simulink model "model"  (R2019b)
settings: Solver=VariableStepAuto  StartTime=0.0  StopTime=50  RelTol=1e-3
values from neighbouring files (symbols this model uses):
  k = 1    [FODT.m]
  kp = T_FODT/(2*k*T_o)    [FODT.m]
  T1 = 5    [FODT.m]
  T2 = 0.1    [FODT.m]
  T3 = 0.05    [FODT.m]
  T4 = 0.025    [FODT.m]
  T_zaklocenia = 25    [FODT.m]
  Ti = T_FODT    [FODT.m]
libraries: simulink_extras x4, simulink x1
settings Model: Creator=szymo  LastModifiedBy=szymo
settings SFSimCC: CustomCodeUndefinedFunction=UseInterfaceOnly

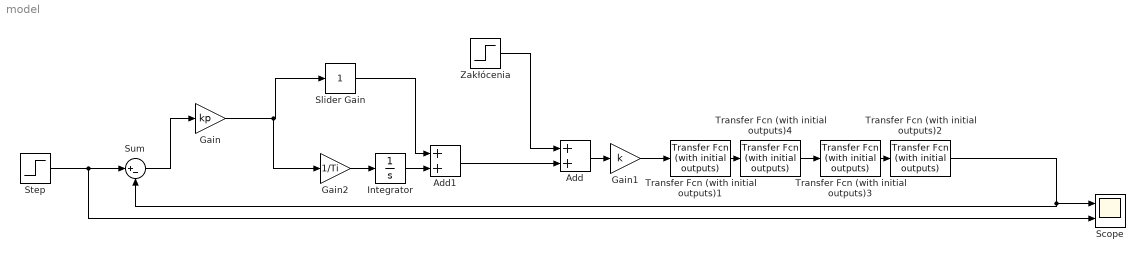
== system model ==
  Add : Sum
  Add1 : Sum
  Gain : Gain  Gain=kp
  Gain1 : Gain  Gain=k
  Gain2 : Gain  Gain=1/Ti
  Integrator : Integrator
  Scope : Scope  NumInputPorts=2
  Slider Gain : simulink/Math Operations/Slider Gain  gain=1  low=0  high=2
  Step : Step  SampleTime=0
  Sum : Sum  Inputs=|+-
  Transfer Fcn (with initial outputs)1 : simulink_extras/Additional Linear/Transfer Fcn (with initial outputs)  N=[1]  D=[T1 1]  Y0=0  U0=0
  Transfer Fcn (with initial outputs)2 : simulink_extras/Additional Linear/Transfer Fcn (with initial outputs)  N=[1]  D="[T4  1]"  Y0=0  U0=0
  Transfer Fcn (with initial outputs)3 : simulink_extras/Additional Linear/Transfer Fcn (with initial outputs)  N=[1]  D="[T3  1]"  Y0=0  U0=0
  Transfer Fcn (with initial outputs)4 : simulink_extras/Additional Linear/Transfer Fcn (with initial outputs)  N=[1]  D=[T2 1]  Y0=0  U0=0
  "Zakłócenia " : Step  Time=T_zaklocenia  After=0.1  SampleTime=0
  wires:
  Step/1 -> Scope/2, Sum/1
  Sum/1 -> Gain/1
  Add1/1 -> Add/2
  Add/1 -> Gain1/1
  Transfer Fcn (with initial outputs)2/1 -> Sum/2, Scope/1
  Gain/1 -> Gain2/1, Slider Gain/1
  Gain2/1 -> Integrator/1
  Integrator/1 -> Add1/2
  Slider Gain/1 -> Add1/1
  Gain1/1 -> Transfer Fcn (with initial outputs)1/1
  Transfer Fcn (with initial outputs)1/1 -> Transfer Fcn (with initial outputs)4/1
  Transfer Fcn (with initial outputs)4/1 -> Transfer Fcn (with initial outputs)3/1
  Transfer Fcn (with initial outputs)3/1 -> Transfer Fcn (with initial outputs)2/1
  "Zakłócenia "/1 -> Add/1
